simulink model "ejercicio"  (Simulink 5.0)
settings: Solver=ode45  StartTime=0.0  StopTime=25  RelTol=1e-3
undefined symbols (not defined in the file): ur
libraries: simulink_extras x1
settings Model: LastModifiedBy=-

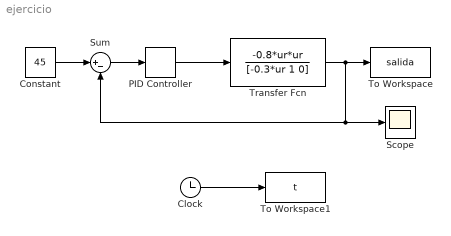
== system ejercicio ==
  Clock : Clock
      settings: Decimation=10
  Constant : Constant  Value=45
  PID Controller : simulink_extras/Additional Linear/PID Controller  P=2.5  I=0  D=3.9
  Scope : Scope
  Sum : Sum  Inputs=|+-  SaturateOnIntegerOverflow=on
  To Workspace : ToWorkspace  VariableName=salida  SampleTime=-1  SaveFormat=Array
  To Workspace1 : ToWorkspace  VariableName=t  SampleTime=-1  SaveFormat=Array
  Transfer Fcn : TransferFcn  Numerator=-0.8*ur*ur  Denominator=[-0.3*ur 1 0]
  wires:
  Constant/1 -> Sum/1
  Sum/1 -> PID Controller/1
  PID Controller/1 -> Transfer Fcn/1
  Transfer Fcn/1 -> To Workspace/1, Scope/1, Sum/2
  Clock/1 -> To Workspace1/1
